simulink model "two_fsk"  (R2018b)
settings: Solver=VariableStepAuto  StartTime=0.0  StopTime=0.1  RelTol=1e-3
libraries: dsparch4 x4, commchan3 x1, commrandsrc3 x1
settings Model: Creator=86138  LastModifiedBy=86138

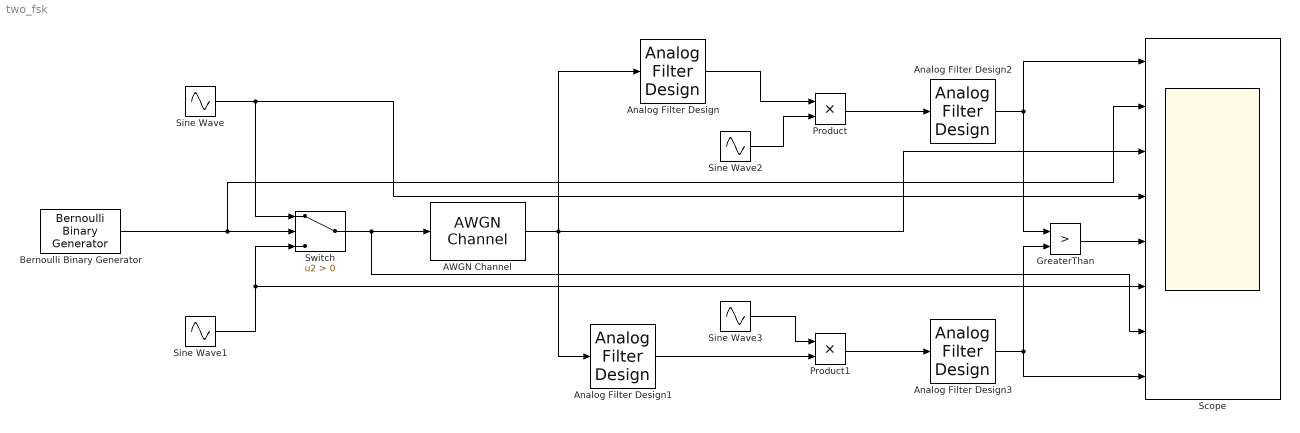
== system two_fsk ==
  AWGN Channel : commchan3/AWGN Channel  InputProcessing=Columns as channels (frame based)  seed=999  noiseMode="Signal to noise ratio  (SNR)"  EbNodB=10  EsNodB=10  SNRdB=10  bitsPerSym=1  Ps=1  Tsym=1  variance=1
  Analog Filter Design : dsparch4/Analog Filter Design  method=Butterworth  filttype=Bandpass  N=8  Wlo=2*pi*10000*985  Whi=2*pi*10000*1015  Rp=2  Rs=40
  Analog Filter Design1 : dsparch4/Analog Filter Design  method=Butterworth  filttype=Bandpass  N=8  Wlo=2*pi*10000*1475  Whi=2*pi*10000*1525  Rp=2  Rs=40
  Analog Filter Design2 : dsparch4/Analog Filter Design  method=Butterworth  filttype=Lowpass  N=8  Wlo=2*pi*10020  Whi=80  Rp=2  Rs=40
  Analog Filter Design3 : dsparch4/Analog Filter Design  method=Butterworth  filttype=Lowpass  N=8  Wlo=2*pi*10050  Whi=80  Rp=2  Rs=40
  Bernoulli Binary Generator : commrandsrc3/Bernoulli Binary Generator  ProbabilityOfZero=0.5  SeedSource=Auto  Seed=0  SampleTime=1/10000  SamplesPerFrame=1  OutputDataType=double  SimulateUsing=Interpreted execution
  GreaterThan : RelationalOperator  Operator=>  OutDataTypeStr=boolean  RndMeth=Simplest
  Product : Product
  Product1 : Product
  Scope : Scope  NumInputPorts=8
  Sine Wave : Sin  Frequency=2*pi*10000*1000  SampleTime=0
  Sine Wave1 : Sin  Frequency=2*pi*10000*1500  SampleTime=0
  Sine Wave2 : Sin  Frequency=2*pi*10000*1000  SampleTime=0
  Sine Wave3 : Sin  Frequency=2*pi*10000*1500  SampleTime=0
  Switch : Switch  Criteria=u2 > Threshold
  wires:
  Sine Wave/1 -> Scope/4, Switch/1
  Bernoulli Binary Generator/1 -> Scope/2, Switch/2
  Sine Wave1/1 -> Scope/6, Switch/3
  Switch/1 -> Scope/7, AWGN Channel/1
  AWGN Channel/1 -> Scope/3, Analog Filter Design/1, Analog Filter Design1/1
  Analog Filter Design/1 -> Product/1
  Analog Filter Design1/1 -> Product1/2
  Sine Wave2/1 -> Product/2
  Sine Wave3/1 -> Product1/1
  Product1/1 -> Analog Filter Design3/1
  Product/1 -> Analog Filter Design2/1
  Analog Filter Design2/1 -> GreaterThan/1, Scope/1
  Analog Filter Design3/1 -> GreaterThan/2, Scope/8
  GreaterThan/1 -> Scope/5
